simulink model "ImpulseGen"  (Simulink 8.3)
settings: Solver=ode45  SolverMode=SingleTasking  StartTime=0.0  StopTime=120.0  MaxStep=.05  RelTol=1e-3  AbsTol=1e-6
undefined symbols (not defined in the file): sfunyst
settings Model: Creator=vise  LastModifiedBy=root  ExtModeTrigMode=oneshot  ExtModeArmWhenConnect=off  ExtModeAutoUpdateStatusClock=off
settings DataIOCC: LimitDataPoints=off
settings OptimizationCC: BooleanDataType=off  ExpressionDepthLimit=2147483647  InitFltsAndDblsToZero=on
settings DebuggingCC: SaveWithParameterizedLinksMsg=none  SignalResolutionControl=TryResolveAllWithWarning  SolverPrmCheckMsg=none  MultiTaskDSMMsg=warning  MultiTaskCondExecSysMsg=none  FcnCallInpInsideContextMsg=UseLocalSettings
settings HardwareCC: TargetUnknown=on
settings RTWCC: TemplateMakefile=grt_unix.tmf  IncludeERTFirstTime=on

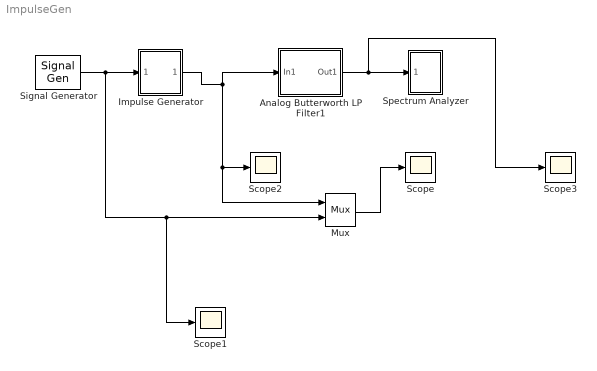
== system ImpulseGen ==
  Analog Butterworth LP Filter1 : Subsystem  mask(buttap){}
      mask help:
      | Analog Butterworth low pass filter.
      |
      | (Requires Signal Processing Toolbox)
      mask init:
      | [z,p,k]=buttap(@2); z=@1*z; p=@1*p; k=real(prod(-p)); [num,den]=zp2tf(z,p,k); w=logspace(log10(@1/10),log10(10*@1),20); h=freqs(num,den,w);
      mask Help: Butterworth low pass filter using MATLAB's butter command.
      mask Display: plot(20*log10(w),20*log10(abs(h)))
  Impulse Generator : Subsystem  mask(D-T interpolator){T=1}
      mask prompts: T "Input sampling period:"
      mask init:
      | L=round(@1/@2);
      mask Display: plot(-10,-10,110,110,[0,50,50,60,60,100],[0,0,80,80,0,0])
  Mux : Mux  Inputs=2
  Scope{,1..3} (4 alike) : Scope
      Scope settings: TickLabels=on  TimeRange=20
      Scope1 settings: TickLabels=on  TimeRange=20
      Scope2 settings: TickLabels=on  TimeRange=20  SaveName=ScopeData2
      Scope3 settings: TickLabels=on  TimeRange=20  SaveName=ScopeData3
  Signal Generator : SignalGenerator  Amplitude=1.000000  Frequency=0.8
  Spectrum Analyzer : Subsystem  LoadFcn=sfunyst([],[],[],'LoadBlock')  mask(Spectrum analyzer.){N=2048, T_s=0.05, plot_period=10}
      mask prompts: N "Number of sample points:"; T_s "Sampling period (sec):"; plot_period "Plotting Period (sec):"
      settings: CopyFcn=sfunyst([],[],[],'CopyBlock')  DeleteFcn=sfunyst([],[],[],'DeleteBlock')
      mask Help: EE438 Lab utility; See Prof. Bouman.
      mask Display: plot(0,0,100,100,[14,91,91,14,14],[86,86,40,40,86],[85,82,80,79,75,67,63,60,57,53,41,36,33,27,24],[49,50,53,50,49,51,54,66,54,50,50,52,81,51,49])
  wires:
  Mux/1 -> Scope/1
  Signal Generator/1 -> Scope1/1, Mux/2, Impulse Generator/1(in_1)
  Impulse Generator/1(out_1) -> Mux/1, Scope2/1, Analog Butterworth LP Filter1/1(In1)
  Analog Butterworth LP Filter1/1(Out1) -> Scope3/1, Spectrum Analyzer/1(input signal)

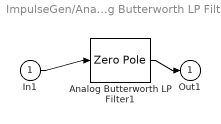
== system ImpulseGen/Analog Butterworth LP Filter1 ==
  In1 : Inport
  Analog Butterworth LP Filter1 : ZeroPole  Zeros=z  Poles=p  Gain=k
  Out1 : Outport
  wires:
  In1/1 -> Analog Butterworth LP Filter1/1
  Analog Butterworth LP Filter1/1 -> Out1/1

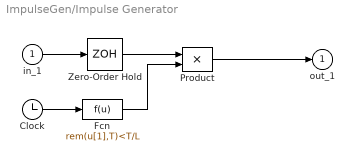
== system ImpulseGen/Impulse Generator ==
  in_1 : Inport
  Clock : Clock
  Fcn : Fcn  Expr=rem(u[1],T)<T/L
  Product : Product  SaturateOnIntegerOverflow=on  RndMeth=Zero  InputSameDT=on  OutDataTypeStr=Inherit: Same as first input
  Zero-Order Hold : ZeroOrderHold  SampleTime=T
  out_1 : Outport  InitialOutput=0
  wires:
  in_1/1 -> Zero-Order Hold/1
  Zero-Order Hold/1 -> Product/1
  Fcn/1 -> Product/2
  Product/1 -> out_1/1
  Clock/1 -> Fcn/1

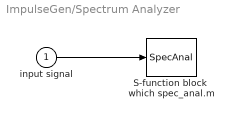
== system ImpulseGen/Spectrum Analyzer ==
  input signal : Inport
  S-function block  which spec_anal.m : S-Function  FunctionName=SpecAnal  Parameters=N,T_s,plot_period  EnableBusSupport=off
  wires:
  input signal/1 -> S-function block  which spec_anal.m/1
